simulink model "Chapter4_GS_and_Flare_controllers_model"  (R2019b)
settings: Solver=VariableStepAuto  StartTime=0.0  StopTime=160  RelTol=1e-3
values from neighbouring files (symbols this model uses):
  alpha = 8.49    [Chapter1_Trim_linearization.m]    (also in Chapter2_OpenLoopAnalysis.m; Chapter3_Pitch_Rate_Command.m; Chapter4_GS_and_Flare_controllers.m)
  altitude = 15000    [Chapter1_Trim_linearization.m]    (also in Chapter2_OpenLoopAnalysis.m = 30000; Chapter3_Pitch_Rate_Command.m = 30000; Chapter4_GS_and_Flare_controllers.m = 5000)
  As = mat_lo([3 7 8 5 11], [3 7 8 5 11])    [Chapter4_GS_and_Flare_controllers.m]
  Bs = mat_lo([3 7 8 5 11], [14 13])    [Chapter4_GS_and_Flare_controllers.m]
  Cs = eye(5)    [Chapter4_GS_and_Flare_controllers.m]
  Ds = zeros(5,2)    [Chapter4_GS_and_Flare_controllers.m]
  pitcha = xu_lo(5)*180/pi    [Chapter4_GS_and_Flare_controllers.m]
  rhflare = hflare+2.5*tau    [Chapter4_GS_and_Flare_controllers.m]
  velocity = 500    [Chapter1_Trim_linearization.m]    (also in Chapter2_OpenLoopAnalysis.m = 600; Chapter3_Pitch_Rate_Command.m = 182.88; Chapter4_GS_and_Flare_controllers.m = 300)
libraries: simulink x5
settings Model: Creator=Luc Kloosterman  LastModifiedBy=Luc Kloosterman

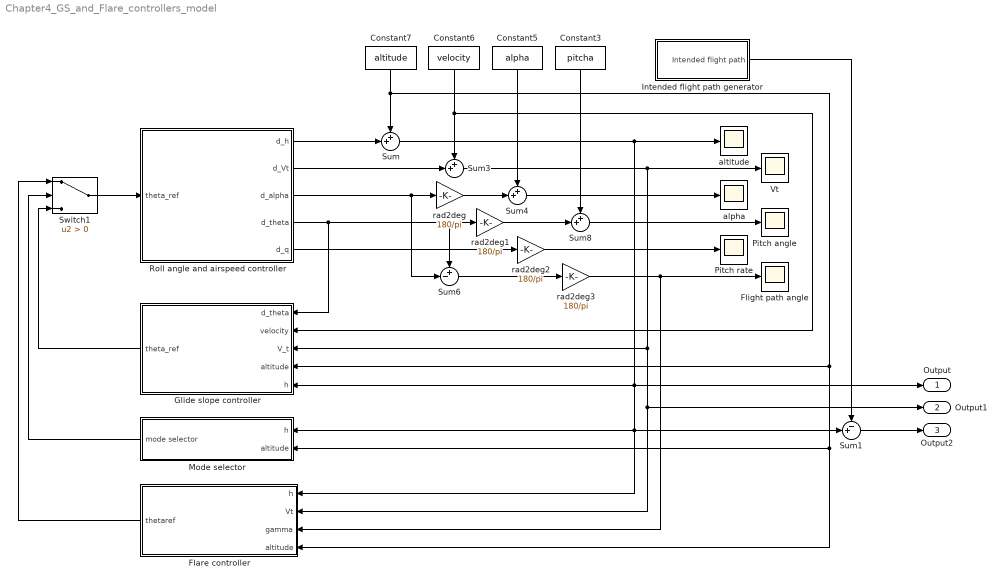
== system Chapter4_GS_and_Flare_controllers_model ==
  Constant3 : Constant  Value=pitcha
  Constant5 : Constant  Value=alpha
  Constant6 : Constant  Value=velocity
  Constant7 : Constant  Value=altitude
  Flare controller : Subsystem
  Flight path angle : Scope
  Glide slope controller : Subsystem
  Intended flight path generator : Subsystem
  Mode selector : Subsystem
  Pitch angle : Scope
  Pitch rate : Scope
  Roll angle and airspeed controller : Subsystem
  Sum{,3..4,8} (4 alike) : Sum  Inputs=++|
  Sum1 : Sum  Inputs=-+|
  Sum6 : Sum  Inputs=+-|
  Switch1 : Switch  Criteria=u2 > Threshold
  Vt : Scope
  alpha : Scope
  altitude : Scope
  rad2deg{,1..3} (4 alike) : Gain  Gain=180/pi
  Output : Outport
  Output1 : Outport  Port=2
  Output2 : Outport  Port=3
  wires:
  Sum4/1 -> alpha/1
  rad2deg1/1 -> Sum8/2
  rad2deg/1 -> Sum4/2
  rad2deg2/1 -> Pitch rate/1
  Sum8/1 -> Pitch angle/1
  Sum6/1 -> rad2deg3/1
  rad2deg3/1 -> Flight path angle/1, Flare controller/3(gamma)
  Flare controller/1(thetaref) -> Switch1/1
  Mode selector/1(mode selector) -> Switch1/2
  Switch1/1 -> Roll angle and airspeed controller/1(theta_ref)
  Roll angle and airspeed controller/1(d_h) -> Sum/2
  Roll angle and airspeed controller/2(d_Vt) -> Sum3/2
  Roll angle and airspeed controller/3(d_alpha) -> Sum6/2, rad2deg/1
  Roll angle and airspeed controller/4(d_theta) -> Glide slope controller/1(d_theta), rad2deg1/1, Sum6/1
  Roll angle and airspeed controller/5(d_q) -> rad2deg2/1
  Glide slope controller/1(theta_ref) -> Switch1/3
  Constant7/1 -> Sum/1, Glide slope controller/4(altitude), Mode selector/2(altitude), Flare controller/4(altitude)
  Constant6/1 -> Glide slope controller/2(velocity), Sum3/1
  Constant5/1 -> Sum4/1
  Constant3/1 -> Sum8/1
  Sum3/1 -> Vt/1, Output1/1, Flare controller/2(Vt), Glide slope controller/3(V_t)
  Sum/1 -> altitude/1, Output/1, Sum1/2, Flare controller/1(h), Mode selector/1(h), Glide slope controller/5(h)
  Intended flight path generator/1(Intended flight path) -> Sum1/1
  Sum1/1 -> Output2/1

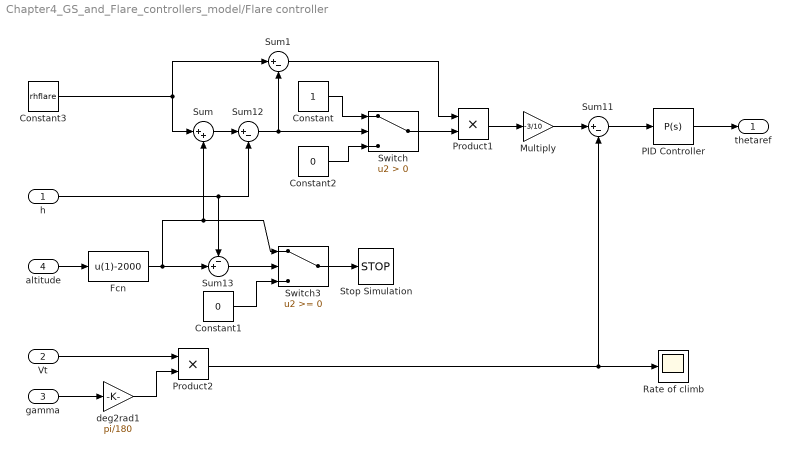
== system Chapter4_GS_and_Flare_controllers_model/Flare controller ==
  h : Inport
  Vt : Inport  Port=2
  gamma : Inport  Port=3
  altitude : Inport  Port=4
  Constant : Constant
  Constant1 : Constant  Value=0
  Constant2 : Constant  Value=0
  Constant3 : Constant  Value=rhflare
  Fcn : Fcn  Expr=u(1)-2000
  Multiply : Gain  Gain=-3/10
  PID Controller : simulink/Continuous/PID Controller  Controller=P  Form=Parallel  TimeDomain=Continuous-time  SampleTime=-1  IntegratorMethod=Forward Euler  FilterMethod=Forward Euler  ControllerParametersSource=internal  P=0.00051045  I=1  D=0  UseFilter=on  N=100  TunerSelectOption=Transfer Function Based (PID Tuner App)  InitialConditionSource=internal  InitialConditionForIntegrator=0  InitialConditionForFilter=0  DifferentiatorICPrevScaledInput=0  ExternalReset=none  TrackingMode=off  Kt=1  LimitOutput=off  UpperSaturationLimit=inf  LowerSaturationLimit=-inf  LinearizeAsGain=on  AntiWindupMode=none  Kb=1  POutMin=[]  POutMax=[]  IOutMin=[]  IOutMax=[]  DOutMin=[]  DOutMax=[]  NOutMin=[]  NOutMax=[]  SumOutMin=[]  SumOutMax=[]  SaturationOutMin=[]  SaturationOutMax=[]  PParamMin=[]  PParamMax=[]  IParamMin=[]  IParamMax=[]  DParamMin=[]  DParamMax=[]  NParamMin=[]  NParamMax=[]  KbParamMin=[]  KbParamMax=[]  KtParamMin=[]  KtParamMax=[]  KbOutMin=[]  KbOutMax=[]  KtOutMin=[]  KtOutMax=[]  IntegratorOutMin=[]  IntegratorOutMax=[]  FilterOutMin=[]  FilterOutMax=[]  SumI1OutMin=[]  SumI1OutMax=[]  SumI2OutMin=[]  SumI2OutMax=[]  SumI3OutMin=[]  SumI3OutMax=[]  SumI4OutMin=[]  SumI4OutMax=[]  SumDOutMin=[]  SumDOutMax=[]  DifferentiatorOutMin=[]  DifferentiatorOutMax=[]  FilterDiffOutCoefMin=[]  FilterDiffOutCoefMax=[]  ReciprocalOutMin=[]  ReciprocalOutMax=[]  SumDenOutMin=[]  SumDenOutMax=[]  SumNumOutMin=[]  SumNumOutMax=[]  DivideOutMin=[]  DivideOutMax=[]  IntegratorContinuousStateAttributes=''  IntegratorStateMustResolveToSignalObject=off  IntegratorRTWStateStorageClass=Auto  FilterContinuousStateAttributes=''  FilterStateMustResolveToSignalObject=off  FilterRTWStateStorageClass=Auto  ParallelPVariant=InternalParameters  IdealPVariant=Disabled  IVariant=Disabled  DVariant=Disabled  IntegratorVariant=Disabled  SatVariant=Disabled  AWVariant=Disabled  PCopyVariant=Disabled  TRVariant=Disabled  FdbkBlocksVariant=Forward  IdealPFdbkVariant=Disabled  SatFdbkVariant=Disabled  DerivativeFilterVariant=Disabled  NVariant=Disabled  NCopyVariant=Disabled_SignalSpec  FilterICVariant=Disabled  IntegratorICVariant=Disabled  ExternalResetVariant=Disabled  TRSumVariant=Passthrough  SumFdbkVariant=Disabled  SumVariant=Passthrough_P
  Product1 : Product
  Product2 : Product
  Rate of climb : Scope
  Stop Simulation : Stop
  Sum : Sum  Inputs=|++
  Sum1 : Sum  Inputs=|+-
  Sum11 : Sum  Inputs=|+-
  Sum12 : Sum  Inputs=|+-
  Sum13 : Sum  Inputs=-+|
  Switch : Switch  Criteria=u2 > Threshold
  Switch3 : Switch
  deg2rad1 : Gain  Gain=pi/180
  thetaref : Outport
  wires:
  altitude/1 -> Fcn/1
  h/1 -> Sum12/2, Sum13/1
  Fcn/1 -> Sum/2, Switch3/1, Sum13/2
  Constant1/1 -> Switch3/3
  Switch3/1 -> Stop Simulation/1
  Sum/1 -> Sum12/1
  Sum12/1 -> Sum1/2, Switch/2
  Constant/1 -> Switch/1
  Constant2/1 -> Switch/3
  Sum1/1 -> Product1/1
  Switch/1 -> Product1/2
  Product1/1 -> Multiply/1
  Multiply/1 -> Sum11/1
  Sum11/1 -> PID Controller/1
  PID Controller/1 -> thetaref/1
  gamma/1 -> deg2rad1/1
  deg2rad1/1 -> Product2/2
  Vt/1 -> Product2/1
  Product2/1 -> Rate of climb/1, Sum11/2
  Sum13/1 -> Switch3/2
  Constant3/1 -> Sum1/1, Sum/1

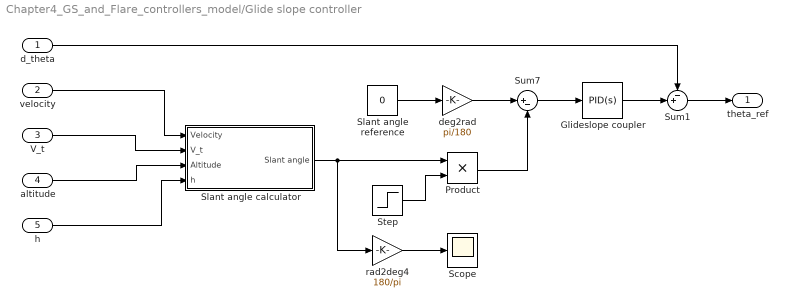
== system Chapter4_GS_and_Flare_controllers_model/Glide slope controller ==
  d_theta : Inport
  velocity : Inport  Port=2
  V_t : Inport  Port=3
  altitude : Inport  Port=4
  h : Inport  Port=5
  Glideslope coupler : simulink/Continuous/PID Controller  Controller=PID  Form=Parallel  TimeDomain=Continuous-time  SampleTime=-1  IntegratorMethod=Forward Euler  FilterMethod=Forward Euler  ControllerParametersSource=internal  P=-55  I=-5  D=5  UseFilter=on  N=0.00395450868065541  TunerSelectOption=Transfer Function Based (PID Tuner App)  InitialConditionSource=internal  InitialConditionForIntegrator=0  InitialConditionForFilter=0  DifferentiatorICPrevScaledInput=0  ExternalReset=none  TrackingMode=off  Kt=1  LimitOutput=off  UpperSaturationLimit=inf  LowerSaturationLimit=-inf  LinearizeAsGain=on  AntiWindupMode=none  Kb=1  POutMin=[]  POutMax=[]  IOutMin=[]  IOutMax=[]  DOutMin=[]  DOutMax=[]  NOutMin=[]  NOutMax=[]  SumOutMin=[]  SumOutMax=[]  SaturationOutMin=[]  SaturationOutMax=[]  PParamMin=[]  PParamMax=[]  IParamMin=[]  IParamMax=[]  DParamMin=[]  DParamMax=[]  NParamMin=[]  NParamMax=[]  KbParamMin=[]  KbParamMax=[]  KtParamMin=[]  KtParamMax=[]  KbOutMin=[]  KbOutMax=[]  KtOutMin=[]  KtOutMax=[]  IntegratorOutMin=[]  IntegratorOutMax=[]  FilterOutMin=[]  FilterOutMax=[]  SumI1OutMin=[]  SumI1OutMax=[]  SumI2OutMin=[]  SumI2OutMax=[]  SumI3OutMin=[]  SumI3OutMax=[]  SumI4OutMin=[]  SumI4OutMax=[]  SumDOutMin=[]  SumDOutMax=[]  DifferentiatorOutMin=[]  DifferentiatorOutMax=[]  FilterDiffOutCoefMin=[]  FilterDiffOutCoefMax=[]  ReciprocalOutMin=[]  ReciprocalOutMax=[]  SumDenOutMin=[]  SumDenOutMax=[]  SumNumOutMin=[]  SumNumOutMax=[]  DivideOutMin=[]  DivideOutMax=[]  IntegratorContinuousStateAttributes=''  IntegratorStateMustResolveToSignalObject=off  IntegratorRTWStateStorageClass=Auto  FilterContinuousStateAttributes=''  FilterStateMustResolveToSignalObject=off  FilterRTWStateStorageClass=Auto  ParallelPVariant=InternalParameters  IdealPVariant=Disabled  IVariant=InternalParameters  DVariant=InternalParameters  IntegratorVariant=Continuous  SatVariant=Disabled  AWVariant=Passthrough  PCopyVariant=Disabled  TRVariant=Disabled  FdbkBlocksVariant=Forward  IdealPFdbkVariant=Disabled  SatFdbkVariant=Disabled  DerivativeFilterVariant=ContFilter  NVariant=InternalParameters  NCopyVariant=Disabled  FilterICVariant=InternalICsFilter  IntegratorICVariant=InternalICs  ExternalResetVariant=Disabled  TRSumVariant=Passthrough  SumFdbkVariant=Disabled  SumVariant=Sum_PID
  Product : Product
  Scope : Scope
  Slant angle calculator : Subsystem
  Slant angle reference : Constant  Value=0
  Step : Step  Time=9.6  SampleTime=0
  Sum1 : Sum  Inputs=-+|
  Sum7 : Sum  Inputs=|+-
  deg2rad : Gain  Gain=pi/180
  rad2deg4 : Gain  Gain=180/pi
  theta_ref : Outport
  wires:
  velocity/1 -> Slant angle calculator/1(Velocity)
  V_t/1 -> Slant angle calculator/2(V_t)
  altitude/1 -> Slant angle calculator/3(Altitude)
  h/1 -> Slant angle calculator/4(h)
  rad2deg4/1 -> Scope/1
  Step/1 -> Product/2
  Slant angle calculator/1(Slant angle) -> Product/1, rad2deg4/1
  Sum7/1 -> Glideslope coupler/1
  Slant angle reference/1 -> deg2rad/1
  deg2rad/1 -> Sum7/1
  Product/1 -> Sum7/2
  Glideslope coupler/1 -> Sum1/2
  Sum1/1 -> theta_ref/1
  d_theta/1 -> Sum1/1

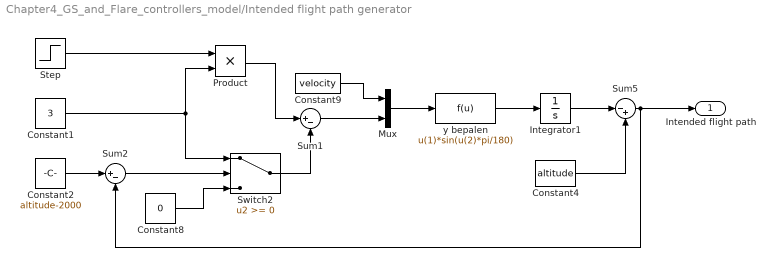
== system Chapter4_GS_and_Flare_controllers_model/Intended flight path generator ==
  Constant1 : Constant  Value=3
  Constant2 : Constant  Value=altitude-2000
  Constant4 : Constant  Value=altitude
  Constant8 : Constant  Value=0
  Constant9 : Constant  Value=velocity
  Integrator1 : Integrator
  Mux : Mux  Inputs=2
  Product : Product
  Step : Step  Time=10  SampleTime=0
  Sum1 : Sum  Inputs=|+-
  Sum2 : Sum  Inputs=|+-
  Sum5 : Sum  Inputs=|-+
  Switch2 : Switch
  y bepalen : Fcn  Expr=u(1)*sin(u(2)*pi/180)
  Intended flight path : Outport
  wires:
  Product/1 -> Sum1/1
  Constant8/1 -> Switch2/3
  Constant9/1 -> Mux/1
  Constant1/1 -> Switch2/1, Product/2
  Switch2/1 -> Sum1/2
  y bepalen/1 -> Integrator1/1
  Sum1/1 -> Mux/2
  Integrator1/1 -> Sum5/1
  Mux/1 -> y bepalen/1
  Constant4/1 -> Sum5/2
  Sum5/1 -> Intended flight path/1, Sum2/2
  Sum2/1 -> Switch2/2
  Constant2/1 -> Sum2/1
  Step/1 -> Product/1

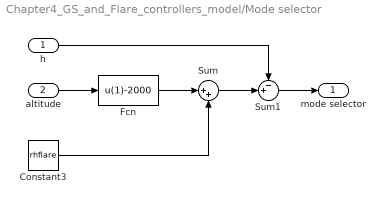
== system Chapter4_GS_and_Flare_controllers_model/Mode selector ==
  h : Inport
  altitude : Inport  Port=2
  Constant3 : Constant  Value=rhflare
  Fcn : Fcn  Expr=u(1)-2000
  Sum : Sum  Inputs=|++
  Sum1 : Sum  Inputs=-+|
  mode selector : Outport
  wires:
  altitude/1 -> Fcn/1
  Constant3/1 -> Sum/2
  Fcn/1 -> Sum/1
  Sum1/1 -> mode selector/1
  Sum/1 -> Sum1/2
  h/1 -> Sum1/1

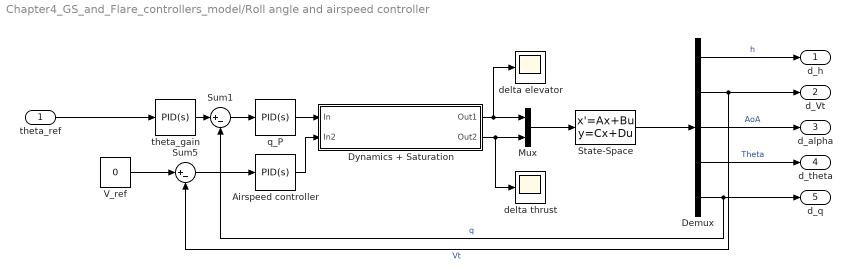
== system Chapter4_GS_and_Flare_controllers_model/Roll angle and airspeed controller ==
  theta_ref : Inport
  " V_ref" : Constant  Value=0
  Airspeed controller : simulink/Continuous/PID Controller  Controller=PID  Form=Parallel  TimeDomain=Continuous-time  SampleTime=-1  IntegratorMethod=Forward Euler  FilterMethod=Forward Euler  ControllerParametersSource=internal  P=2000  I=50  D=1500  UseFilter=on  N=3.67106722852545  TunerSelectOption=Transfer Function Based (PID Tuner App)  InitialConditionSource=internal  InitialConditionForIntegrator=0  InitialConditionForFilter=0  DifferentiatorICPrevScaledInput=0  ExternalReset=none  TrackingMode=off  Kt=1  LimitOutput=off  UpperSaturationLimit=inf  LowerSaturationLimit=-inf  LinearizeAsGain=on  AntiWindupMode=none  Kb=1  POutMin=[]  POutMax=[]  IOutMin=[]  IOutMax=[]  DOutMin=[]  DOutMax=[]  NOutMin=[]  NOutMax=[]  SumOutMin=[]  SumOutMax=[]  SaturationOutMin=[]  SaturationOutMax=[]  PParamMin=[]  PParamMax=[]  IParamMin=[]  IParamMax=[]  DParamMin=[]  DParamMax=[]  NParamMin=[]  NParamMax=[]  KbParamMin=[]  KbParamMax=[]  KtParamMin=[]  KtParamMax=[]  KbOutMin=[]  KbOutMax=[]  KtOutMin=[]  KtOutMax=[]  IntegratorOutMin=[]  IntegratorOutMax=[]  FilterOutMin=[]  FilterOutMax=[]  SumI1OutMin=[]  SumI1OutMax=[]  SumI2OutMin=[]  SumI2OutMax=[]  SumI3OutMin=[]  SumI3OutMax=[]  SumI4OutMin=[]  SumI4OutMax=[]  SumDOutMin=[]  SumDOutMax=[]  DifferentiatorOutMin=[]  DifferentiatorOutMax=[]  FilterDiffOutCoefMin=[]  FilterDiffOutCoefMax=[]  ReciprocalOutMin=[]  ReciprocalOutMax=[]  SumDenOutMin=[]  SumDenOutMax=[]  SumNumOutMin=[]  SumNumOutMax=[]  DivideOutMin=[]  DivideOutMax=[]  IntegratorContinuousStateAttributes=''  IntegratorStateMustResolveToSignalObject=off  IntegratorRTWStateStorageClass=Auto  FilterContinuousStateAttributes=''  FilterStateMustResolveToSignalObject=off  FilterRTWStateStorageClass=Auto  ParallelPVariant=InternalParameters  IdealPVariant=Disabled  IVariant=InternalParameters  DVariant=InternalParameters  IntegratorVariant=Continuous  SatVariant=Disabled  AWVariant=Passthrough  PCopyVariant=Disabled  TRVariant=Disabled  FdbkBlocksVariant=Forward  IdealPFdbkVariant=Disabled  SatFdbkVariant=Disabled  DerivativeFilterVariant=ContFilter  NVariant=InternalParameters  NCopyVariant=Disabled  FilterICVariant=InternalICsFilter  IntegratorICVariant=InternalICs  ExternalResetVariant=Disabled  TRSumVariant=Passthrough  SumFdbkVariant=Disabled  SumVariant=Sum_PID
  Demux : Demux  Outputs=5
  Dynamics + Saturation : Subsystem
  Mux : Mux  Inputs=2
  State-Space : StateSpace  A=As  B=Bs  C=Cs  D=Ds  InitialCondition=0
  Sum1 : Sum  Inputs=|+-
  Sum5 : Sum  Inputs=|+-
  delta elevator : Scope
  delta thrust : Scope
  q_P : simulink/Continuous/PID Controller  Controller=PID  Form=Parallel  TimeDomain=Continuous-time  SampleTime=-1  IntegratorMethod=Forward Euler  FilterMethod=Forward Euler  ControllerParametersSource=internal  P=-509.387552005556  I=-1672.89207194643  D=-25.6166684441567  UseFilter=on  N=3796.0293831992  TunerSelectOption=Transfer Function Based (PID Tuner App)  InitialConditionSource=internal  InitialConditionForIntegrator=0  InitialConditionForFilter=0  DifferentiatorICPrevScaledInput=0  ExternalReset=none  TrackingMode=off  Kt=1  LimitOutput=off  UpperSaturationLimit=inf  LowerSaturationLimit=-inf  LinearizeAsGain=on  AntiWindupMode=none  Kb=1  POutMin=[]  POutMax=[]  IOutMin=[]  IOutMax=[]  DOutMin=[]  DOutMax=[]  NOutMin=[]  NOutMax=[]  SumOutMin=[]  SumOutMax=[]  SaturationOutMin=[]  SaturationOutMax=[]  PParamMin=[]  PParamMax=[]  IParamMin=[]  IParamMax=[]  DParamMin=[]  DParamMax=[]  NParamMin=[]  NParamMax=[]  KbParamMin=[]  KbParamMax=[]  KtParamMin=[]  KtParamMax=[]  KbOutMin=[]  KbOutMax=[]  KtOutMin=[]  KtOutMax=[]  IntegratorOutMin=[]  IntegratorOutMax=[]  FilterOutMin=[]  FilterOutMax=[]  SumI1OutMin=[]  SumI1OutMax=[]  SumI2OutMin=[]  SumI2OutMax=[]  SumI3OutMin=[]  SumI3OutMax=[]  SumI4OutMin=[]  SumI4OutMax=[]  SumDOutMin=[]  SumDOutMax=[]  DifferentiatorOutMin=[]  DifferentiatorOutMax=[]  FilterDiffOutCoefMin=[]  FilterDiffOutCoefMax=[]  ReciprocalOutMin=[]  ReciprocalOutMax=[]  SumDenOutMin=[]  SumDenOutMax=[]  SumNumOutMin=[]  SumNumOutMax=[]  DivideOutMin=[]  DivideOutMax=[]  IntegratorContinuousStateAttributes=''  IntegratorStateMustResolveToSignalObject=off  IntegratorRTWStateStorageClass=Auto  FilterContinuousStateAttributes=''  FilterStateMustResolveToSignalObject=off  FilterRTWStateStorageClass=Auto  ParallelPVariant=InternalParameters  IdealPVariant=Disabled  IVariant=InternalParameters  DVariant=InternalParameters  IntegratorVariant=Continuous  SatVariant=Disabled  AWVariant=Passthrough  PCopyVariant=Disabled  TRVariant=Disabled  FdbkBlocksVariant=Forward  IdealPFdbkVariant=Disabled  SatFdbkVariant=Disabled  DerivativeFilterVariant=ContFilter  NVariant=InternalParameters  NCopyVariant=Disabled  FilterICVariant=InternalICsFilter  IntegratorICVariant=InternalICs  ExternalResetVariant=Disabled  TRSumVariant=Passthrough  SumFdbkVariant=Disabled  SumVariant=Sum_PID
  theta_gain : simulink/Continuous/PID Controller  Controller=PID  Form=Parallel  TimeDomain=Continuous-time  SampleTime=-1  IntegratorMethod=Forward Euler  FilterMethod=Forward Euler  ControllerParametersSource=internal  P=3.35835507161287  I=1.39931031411675  D=1.00753606070998  UseFilter=on  N=321.707950566768  TunerSelectOption=Transfer Function Based (PID Tuner App)  InitialConditionSource=internal  InitialConditionForIntegrator=0  InitialConditionForFilter=0  DifferentiatorICPrevScaledInput=0  ExternalReset=none  TrackingMode=off  Kt=1  LimitOutput=off  UpperSaturationLimit=inf  LowerSaturationLimit=-inf  LinearizeAsGain=on  AntiWindupMode=none  Kb=1  POutMin=[]  POutMax=[]  IOutMin=[]  IOutMax=[]  DOutMin=[]  DOutMax=[]  NOutMin=[]  NOutMax=[]  SumOutMin=[]  SumOutMax=[]  SaturationOutMin=[]  SaturationOutMax=[]  PParamMin=[]  PParamMax=[]  IParamMin=[]  IParamMax=[]  DParamMin=[]  DParamMax=[]  NParamMin=[]  NParamMax=[]  KbParamMin=[]  KbParamMax=[]  KtParamMin=[]  KtParamMax=[]  KbOutMin=[]  KbOutMax=[]  KtOutMin=[]  KtOutMax=[]  IntegratorOutMin=[]  IntegratorOutMax=[]  FilterOutMin=[]  FilterOutMax=[]  SumI1OutMin=[]  SumI1OutMax=[]  SumI2OutMin=[]  SumI2OutMax=[]  SumI3OutMin=[]  SumI3OutMax=[]  SumI4OutMin=[]  SumI4OutMax=[]  SumDOutMin=[]  SumDOutMax=[]  DifferentiatorOutMin=[]  DifferentiatorOutMax=[]  FilterDiffOutCoefMin=[]  FilterDiffOutCoefMax=[]  ReciprocalOutMin=[]  ReciprocalOutMax=[]  SumDenOutMin=[]  SumDenOutMax=[]  SumNumOutMin=[]  SumNumOutMax=[]  DivideOutMin=[]  DivideOutMax=[]  IntegratorContinuousStateAttributes=''  IntegratorStateMustResolveToSignalObject=off  IntegratorRTWStateStorageClass=Auto  FilterContinuousStateAttributes=''  FilterStateMustResolveToSignalObject=off  FilterRTWStateStorageClass=Auto  ParallelPVariant=InternalParameters  IdealPVariant=Disabled  IVariant=InternalParameters  DVariant=InternalParameters  IntegratorVariant=Continuous  SatVariant=Disabled  AWVariant=Passthrough  PCopyVariant=Disabled  TRVariant=Disabled  FdbkBlocksVariant=Forward  IdealPFdbkVariant=Disabled  SatFdbkVariant=Disabled  DerivativeFilterVariant=ContFilter  NVariant=InternalParameters  NCopyVariant=Disabled  FilterICVariant=InternalICsFilter  IntegratorICVariant=InternalICs  ExternalResetVariant=Disabled  TRSumVariant=Passthrough  SumFdbkVariant=Disabled  SumVariant=Sum_PID
  d_h : Outport
  d_Vt : Outport  Port=2
  d_alpha : Outport  Port=3
  d_theta : Outport  Port=4
  d_q : Outport  Port=5
  wires:
  " V_ref"/1 -> Sum5/1
  theta_ref/1 -> theta_gain/1
  Demux/2 -> d_Vt/1, Sum5/2  "Vt"
  Sum5/1 -> Airspeed controller/1
  theta_gain/1 -> Sum1/1
  Airspeed controller/1 -> Dynamics + Saturation/2(In2)
  Demux/5 -> d_q/1, Sum1/2  "q"
  State-Space/1 -> Demux/1
  Sum1/1 -> q_P/1
  q_P/1 -> Dynamics + Saturation/1("In ")
  Dynamics + Saturation/2(Out2) -> delta thrust/1, Mux/2
  Mux/1 -> State-Space/1
  Demux/1 -> d_h/1  "h"
  Demux/3 -> d_alpha/1  "AoA"
  Demux/4 -> d_theta/1  "Theta"
  Dynamics + Saturation/1(Out1) -> Mux/1, delta elevator/1

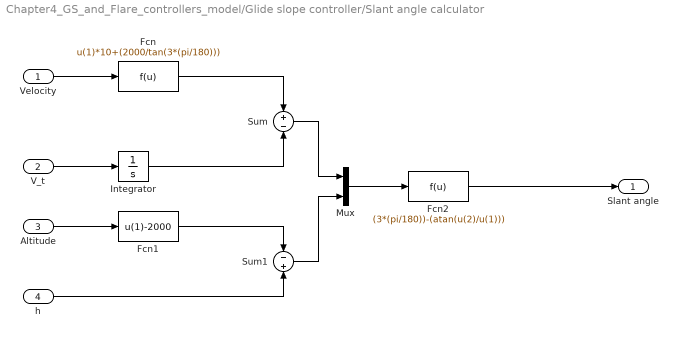
== system Chapter4_GS_and_Flare_controllers_model/Glide slope controller/Slant angle calculator ==
  Velocity : Inport
  V_t : Inport  Port=2
  Altitude : Inport  Port=3
  h : Inport  Port=4
  Fcn : Fcn  Expr=u(1)*10+(2000/tan(3*(pi/180)))
  Fcn1 : Fcn  Expr=u(1)-2000
  Fcn2 : Fcn  Expr=(3*(pi/180))-(atan(u(2)/u(1)))
  Integrator : Integrator
  Mux : Mux  Inputs=2
  Sum : Sum  Inputs=+|-
  Sum1 : Sum  Inputs=-|+
  Slant angle : Outport
  wires:
  Velocity/1 -> Fcn/1
  Altitude/1 -> Fcn1/1
  Fcn/1 -> Sum/1
  Integrator/1 -> Sum/2
  Fcn1/1 -> Sum1/1
  h/1 -> Sum1/2
  Sum1/1 -> Mux/2
  Sum/1 -> Mux/1
  Mux/1 -> Fcn2/1
  Fcn2/1 -> Slant angle/1
  V_t/1 -> Integrator/1

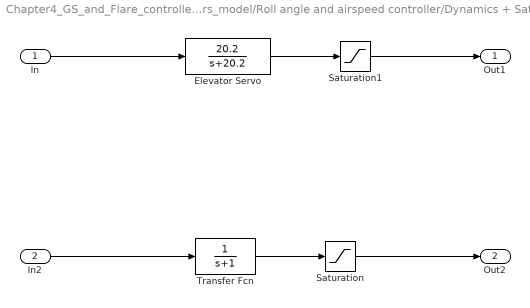
== system Chapter4_GS_and_Flare_controllers_model/Roll angle and airspeed controller/Dynamics + Saturation ==
  "In " : Inport
  In2 : Inport  Port=2
  Elevator Servo : TransferFcn  Numerator=[20.2]  Denominator=[1 20.2]
  Saturation : Saturate  UpperLimit=1.6489e+04  LowerLimit=-1.5106e+03
  Saturation1 : Saturate  UpperLimit=21.2217  LowerLimit=-28.7783
  Transfer Fcn : TransferFcn  Denominator=[1 1]
  Out1 : Outport
  Out2 : Outport  Port=2
  wires:
  Transfer Fcn/1 -> Saturation/1
  Elevator Servo/1 -> Saturation1/1
  "In "/1 -> Elevator Servo/1
  Saturation1/1 -> Out1/1
  In2/1 -> Transfer Fcn/1
  Saturation/1 -> Out2/1
